simulink model "Demo"  (R2021a)
settings: Solver=FixedStepDiscrete  StartTime=0.0  StopTime=10  FixedStep=0.005  RelTol=1e-3  EnableMultiTasking=on
PreLoadFcn:
  | disp(pwd)
PostLoadFcn:
  | c2000demoscallback(1)
undefined symbols (not defined in the file or in its folder): CommandConstEnable, CommandData, FrameData, MailBoxRx, MailBoxTx, SCIAReceivedComplete, StatusConstClose, StatusConstClosed, StatusConstError, StatusConstHoming, StatusConstIdle, StatusConstPaused, StatusConstReady, StatusConstReset, StatusConstRunning, StatusConstStart, StatusConstStopped, StatusData
libraries: simulink x28, c280xlib x19, idelinklib_common x16, c2000lib x1, pid_lib x1, c2833xlib x1
(part 2 of 3)

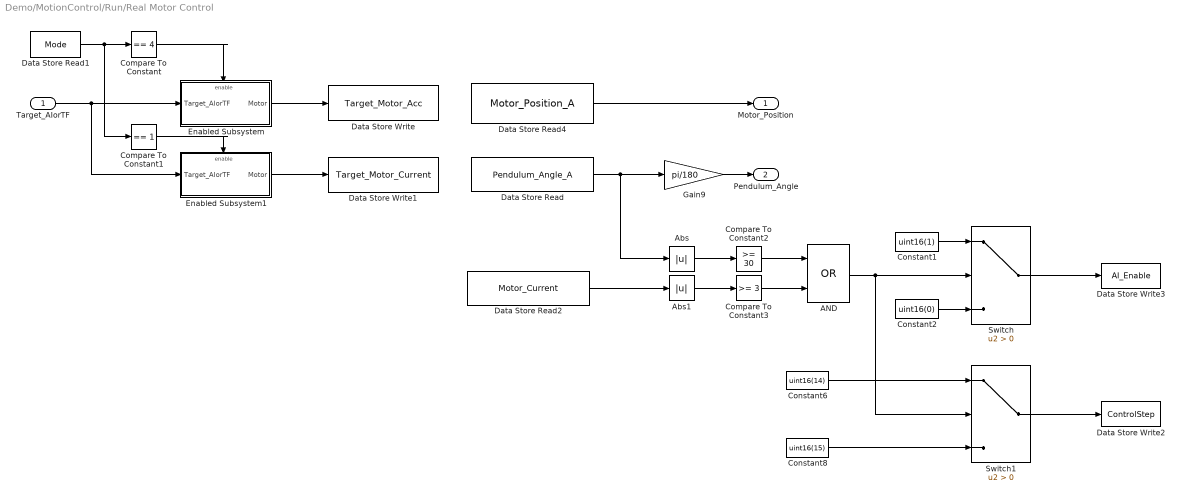
== system Demo/MotionControl/Run/Real Motor Control ==
  Target_AIorTF : Inport
  AND : Logic  Operator=OR  AllPortsSameDT=off  OutDataTypeStr=boolean
  Abs : Abs
  Abs1 : Abs
  Compare To Constant : simulink/Logic and Bit Operations/Compare To Constant  relop===  const=4  OutDataTypeStr=boolean
  Compare To Constant1 : simulink/Logic and Bit Operations/Compare To Constant  relop===  const=1  OutDataTypeStr=boolean
  Compare To Constant2 : simulink/Logic and Bit Operations/Compare To Constant  relop=>=  const=30  OutDataTypeStr=boolean
  Compare To Constant3 : simulink/Logic and Bit Operations/Compare To Constant  relop=>=  const=3  OutDataTypeStr=boolean
  Constant1 : Constant  Value=uint16(1)
  Constant2 : Constant  Value=uint16(0)
  Constant6 : Constant  Value=uint16(14)
  Constant8 : Constant  Value=uint16(15)
  Data Store Read : DataStoreRead  DataStoreName=Pendulum_Angle_A  IndexOptions=Index vector (dialog)  Indices=1  OutputSizes=1
  Data Store Read1 : DataStoreRead  DataStoreName=Mode  IndexOptions=Index vector (dialog)  Indices=1  OutputSizes=1
  Data Store Read2 : DataStoreRead  DataStoreName=Motor_Current  IndexOptions=Index vector (dialog)  Indices=1  OutputSizes=1
  Data Store Read4 : DataStoreRead  DataStoreName=Motor_Position_A  IndexOptions=Index vector (dialog)  Indices=1  OutputSizes=1
  Data Store Write : DataStoreWrite  DataStoreName=Target_Motor_Acc  IndexOptions=Index vector (dialog)  Indices=1  OutputSizes=1
  Data Store Write1 : DataStoreWrite  DataStoreName=Target_Motor_Current  IndexOptions=Index vector (dialog)  Indices=1  OutputSizes=1
  Data Store Write2 : DataStoreWrite  DataStoreName=ControlStep  IndexOptions=Index vector (dialog)  Indices=1  OutputSizes=1
  Data Store Write3 : DataStoreWrite  DataStoreName=AI_Enable  IndexOptions=Index vector (dialog)  Indices=1  OutputSizes=1
  Enabled Subsystem : Subsystem  TreatAsAtomicUnit=on
  Enabled Subsystem1 : Subsystem  TreatAsAtomicUnit=on
  Gain9 : Gain  Gain=pi/180  OutDataTypeStr=double
  Switch : Switch  Criteria=u2 > Threshold
  Switch1 : Switch  Criteria=u2 > Threshold
  Motor_Position : Outport  VectorParamsAs1DForOutWhenUnconnected=off
  Pendulum_Angle : Outport  Port=2  VectorParamsAs1DForOutWhenUnconnected=off
  wires:
  Compare To Constant1/1 -> Enabled Subsystem1/Enable
  Enabled Subsystem1/1(Motor) -> Data Store Write1/1
  Enabled Subsystem/1(Motor) -> Data Store Write/1
  Compare To Constant/1 -> Enabled Subsystem/Enable
  Data Store Read1/1 -> Compare To Constant/1, Compare To Constant1/1
  Target_AIorTF/1 -> Enabled Subsystem/1(Target_AIorTF), Enabled Subsystem1/1(Target_AIorTF)
  Gain9/1 -> Pendulum_Angle/1
  Data Store Read4/1 -> Motor_Position/1
  Compare To Constant2/1 -> AND/1
  Compare To Constant3/1 -> AND/2
  AND/1 -> Switch1/2, Switch/2
  Constant8/1 -> Switch1/3
  Data Store Read2/1 -> Abs1/1
  Abs1/1 -> Compare To Constant3/1
  Constant2/1 -> Switch/3
  Constant6/1 -> Switch1/1
  Abs/1 -> Compare To Constant2/1
  Data Store Read/1 -> Abs/1, Gain9/1
  Switch/1 -> Data Store Write3/1
  Switch1/1 -> Data Store Write2/1
  Constant1/1 -> Switch/1

== system Demo/MotionControl/Start/BG ==
  Action Port : ActionPort  ActionPortLabel=case [ 3 ]:
  BG : Constant  Value=[hex2dec('4742') 0 0 0]  OutDataTypeStr=uint16
  Constant : Constant  Value=uint16(15)  SampleTime=-1
  Data Store Write2 : DataStoreWrite  DataStoreName=ControlStep  IndexOptions=Index vector (dialog)  Indices=1  OutputSizes=1
  eCANA Transmit : Subsystem  TreatAsAtomicUnit=on  mask(eCANA Transimit Blocks){MailBoxTx=1, MailBoxRx=4}
      mask help: eCANA MailBox Transimit
      mask DialogControl ParameterGroup Prompt: Parameter Setting
  wires:
  BG/1 -> eCANA Transmit/1(DataTx)
  Constant/1 -> Data Store Write2/1

== system Demo/MotionControl/Start/MO=1 ==
  Action Port : ActionPort  ActionPortLabel=case [ 1 ]:
  Add Constant : Bias  Bias=uint16(1)
  Data Store Read : DataStoreRead  DataStoreName=ControlStep  IndexOptions=Index vector (dialog)  Indices=1  OutputSizes=1
  Data Store Write1 : DataStoreWrite  DataStoreName=ControlStep  IndexOptions=Index vector (dialog)  Indices=1  OutputSizes=1
  Delay500ms : Subsystem  mask(System Outputs){ShowInLibBrowser=0}
      mask prompts: ShowInLibBrowser "Simulink:masks:CustCodeMaskParam1_MP"
      settings: CopyFcn=cccopyfcn(gcb)  OpenFcn=ccopenfcn('System Outputs Function')
      mask Help: eval('feval(''rtwprivate'',''rtwhelpview'',''rtw_sys_outputs_block'')');
      mask Display: disp('System\nOutputs');
  MO : Constant  Value=[hex2dec('4F4D') 0 1 0]  OutDataTypeStr=uint16
  eCANA Transmit : Subsystem  TreatAsAtomicUnit=on  mask(eCANA Transimit Blocks){MailBoxTx=1, MailBoxRx=4}
      mask help: eCANA MailBox Transimit
      mask DialogControl ParameterGroup Prompt: Parameter Setting
  wires:
  Add Constant/1 -> Data Store Write1/1
  MO/1 -> eCANA Transmit/1(DataTx)
  Data Store Read/1 -> Add Constant/1

== system Demo/MotionControl/Start/UM=1or4 ==
  Action Port : ActionPort  ActionPortLabel=case [ 2 ]:
  Add Constant : Bias  Bias=uint16(1)
  Constant : Constant  Value=hex2dec('4D55')  OutDataTypeStr=uint16
  Constant1 : Constant  Value=uint16(0)
  Constant2 : Constant  Value=uint16(0)
  Constant3 : Constant  Value=uint16(1)
  Constant4 : Constant  Value=uint16(4)
  Data Store Read : DataStoreRead  DataStoreName=ControlStep  IndexOptions=Index vector (dialog)  Indices=1  OutputSizes=1
  Data Store Read1 : DataStoreRead  DataStoreName=CommandData  IndexOptions=Index vector (dialog)  Indices=1  OutputSizes=1
  Data Store Write1 : DataStoreWrite  DataStoreName=ControlStep  IndexOptions=Index vector (dialog)  Indices=1  OutputSizes=1
  Data Store Write2 : DataStoreWrite  DataStoreName=Mode  IndexOptions=Index vector (dialog)  Indices=1  OutputSizes=1
  Mux : Mux
  Selector : Selector  InputPortWidth=8  IndexOptions=Index vector (dialog)  Indices=1  OutputSizes=1
  Switch : Switch  Criteria=u2 > Threshold
  eCANA Transmit : Subsystem  TreatAsAtomicUnit=on  mask(eCANA Transimit Blocks){MailBoxTx=1, MailBoxRx=4}
      mask help: eCANA MailBox Transimit
      mask DialogControl ParameterGroup Prompt: Parameter Setting
  wires:
  Add Constant/1 -> Data Store Write1/1
  Data Store Read/1 -> Add Constant/1
  Constant2/1 -> Mux/4
  Data Store Read1/1 -> Selector/1
  Constant3/1 -> Switch/1
  Constant4/1 -> Switch/3
  Constant/1 -> Mux/1
  Constant1/1 -> Mux/2
  Mux/1 -> eCANA Transmit/1(DataTx)
  Selector/1 -> Switch/2
  Switch/1 -> Data Store Write2/1, Mux/3

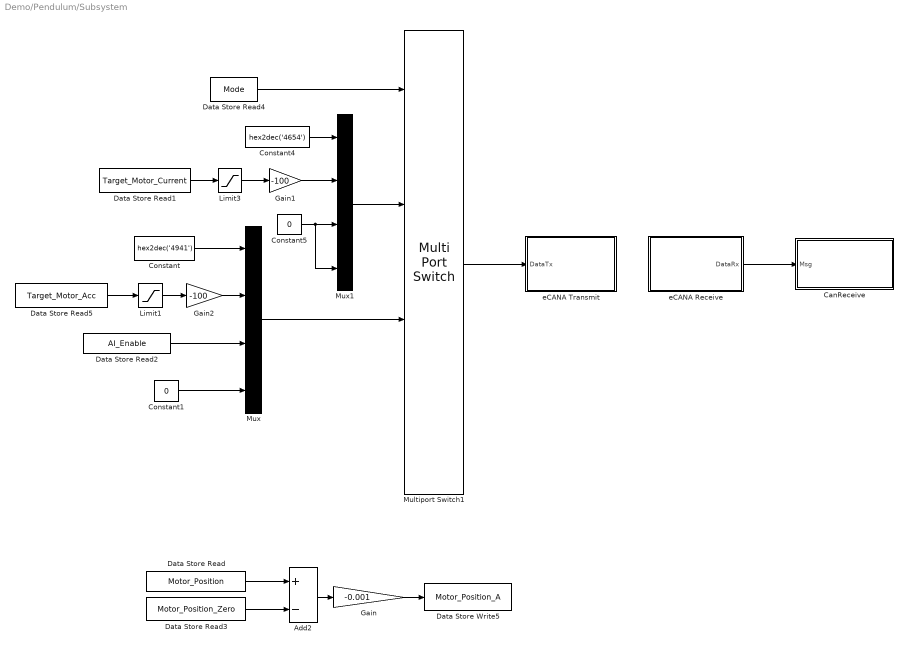
== system Demo/Pendulum/Subsystem ==
  Add2 : Sum  Inputs=+-
  CanReceive : Subsystem  TreatAsAtomicUnit=on
  Constant : Constant  Value=hex2dec('4941')  OutDataTypeStr=uint16
  Constant1 : Constant  Value=0  OutDataTypeStr=uint16
  Constant4 : Constant  Value=hex2dec('4654')  OutDataTypeStr=uint16
  Constant5 : Constant  Value=0  OutDataTypeStr=uint16
  Data Store Read : DataStoreRead  DataStoreName=Motor_Position  IndexOptions=Index vector (dialog)  Indices=1  OutputSizes=1
  Data Store Read1 : DataStoreRead  DataStoreName=Target_Motor_Current  IndexOptions=Index vector (dialog)  Indices=1  OutputSizes=1
  Data Store Read2 : DataStoreRead  DataStoreName=AI_Enable  IndexOptions=Index vector (dialog)  Indices=1  OutputSizes=1
  Data Store Read3 : DataStoreRead  DataStoreName=Motor_Position_Zero  IndexOptions=Index vector (dialog)  Indices=1  OutputSizes=1
  Data Store Read4 : DataStoreRead  DataStoreName=Mode  IndexOptions=Index vector (dialog)  Indices=1  OutputSizes=1
  Data Store Read5 : DataStoreRead  DataStoreName=Target_Motor_Acc  IndexOptions=Index vector (dialog)  Indices=1  OutputSizes=1
  Data Store Write5 : DataStoreWrite  DataStoreName=Motor_Position_A  IndexOptions=Index vector (dialog)  Indices=1  OutputSizes=1
  Gain : Gain  Gain=-0.001
  Gain1 : Gain  Gain=-100  OutDataTypeStr=uint16
  Gain2 : Gain  Gain=-100  OutDataTypeStr=uint16
  Limit1 : Saturate  UpperLimit=300  LowerLimit=-300
  Limit3 : Saturate  UpperLimit=3  LowerLimit=-3
  Multiport Switch1 : MultiPortSwitch  DataPortOrder=Specify indices  DataPortIndices={1,4}  DataPortForDefault=Additional data port  DiagnosticForDefault=None
  Mux : Mux
  Mux1 : Mux
  eCANA Receive : Subsystem  TreatAsAtomicUnit=on  mask(eCANA Transimit Blocks){MailBoxTx=1, MailBoxRx=4}
      mask help: eCANA MailBox Transimit
      mask DialogControl ParameterGroup Prompt: Parameter Setting
  eCANA Transmit : Subsystem  TreatAsAtomicUnit=on  mask(eCANA Transimit Blocks){MailBoxTx=1, MailBoxRx=4}
      mask help: eCANA MailBox Transimit
      mask DialogControl ParameterGroup Prompt: Parameter Setting
  wires:
  Data Store Read1/1 -> Limit3/1
  Data Store Read4/1 -> Multiport Switch1/1
  Constant4/1 -> Mux1/1
  Constant5/1 -> Mux1/4, Mux1/3
  Constant1/1 -> Mux/4
  Constant/1 -> Mux/1
  Data Store Read5/1 -> Limit1/1
  Gain/1 -> Data Store Write5/1
  Data Store Read3/1 -> Add2/2
  Add2/1 -> Gain/1
  Data Store Read/1 -> Add2/1
  Gain2/1 -> Mux/2
  Gain1/1 -> Mux1/2
  Mux/1 -> Multiport Switch1/3
  Mux1/1 -> Multiport Switch1/2
  Multiport Switch1/1 -> eCANA Transmit/1(DataTx)
  eCANA Receive/1(DataRx) -> CanReceive/1(Msg)
  Data Store Read2/1 -> Mux/3
  Limit1/1 -> Gain2/1
  Limit3/1 -> Gain1/1

== system Demo/Pendulum/Subsystem1 ==
  Add : Sum  Inputs=+-
  Data Store Read1 : DataStoreRead  DataStoreName=Pendulum_Angle_Zero  IndexOptions=Index vector (dialog)  Indices=1  OutputSizes=1
  Data Store Write1 : DataStoreWrite  DataStoreName=Pendulum_Angle_A  IndexOptions=Index vector (dialog)  Indices=1  OutputSizes=1
  Data Store Write2 : DataStoreWrite  DataStoreName=Pendulum_Angle  IndexOptions=Index vector (dialog)  Indices=1  OutputSizes=1
  Gain1 : Gain  Gain=360/10000  OutDataTypeStr=double
  eQEP : c280xlib/eQEP  useModule=eQEP1  pcInputmode=Quadrature-count  externalClockrate=2x resolution: Count the rising/falling edge  swapPolarityselection=Counterclockwise  qdfOutputport=off  qapPolarityselection=off  qbpPolarityselection=off  qipPolarityselection=off  qspPolarityselection=off  igatePolarityselection=off  sampleTime=-1  pcOutputport=on  pcMaximumvalue=4294967295  indexInitializationcheck=off  indexInitializationevent=Rising edge  strobeInitializationcheck=off  strobeInitializationevent=Rising edge  softwareInitializationcheck=on  softwareInitializationsource=Set to init value at start up  softwareInitializationmode=on  pcInitialvalue=4294962296  pcResetmode=Reset on the maximum position  ieloutputport=off  indexEventlatch=Rising edge  seloutputport=off  strobeEventlatch=Rising edge  pcefOutputport=off  enableEqepcapture=off  qctmrOutputport=off  qcprdOutputport=off  captureTimerprescaler=128  upEventprescaler=128  overflowErrorflag=off  directionErrorflag=off  captureTimerposition=On position counter read  unitTimerperiod=100000000  captureTimerlatch=off  capturePeriodlatch=off  positionCounterlatch=off  soenPolarityselection=off  spselPolarityselection=Index pin is used for sync output  compareValuesource=Specify via dialog  shadowMode=Load on QPOSCNT=0  compareValue=4294967295  syncOutputwidth=1  polaritySyncoutput=Active high  watchdogEnable=off  watchdogTimer=65535  outport1Datatype=auto  outport2Datatype=int32  outport3Datatype=auto  outport4Datatype=auto  outport5Datatype=auto  outport6Datatype=auto  outport7Datatype=auto  outport8Datatype=auto  outport9Datatype=auto  outport10Datatype=auto  outport11Datatype=auto  outport12Datatype=auto  eqepinterrupt_pce=off  eqepinterrupt_qpe=off  eqepinterrupt_qdc=off  eqepinterrupt_wto=off  eqepinterrupt_pcu=off  eqepinterrupt_pco=off  eqepinterrupt_pcr=off  eqepinterrupt_pcm=off  eqepinterrupt_sel=off  eqepinterrupt_iel=off  eqepinterrupt_uto=off  pheOutputport=off  watchdogOutputport=off  outport13Datatype=auto  outport14Datatype=auto
      settings: SourceProductName=Embedded Coder Support Package for Texas Instruments C2000 Processors
  wires:
  Data Store Read1/1 -> Add/2
  Gain1/1 -> Add/1, Data Store Write2/1
  eQEP/1 -> Gain1/1
  Add/1 -> Data Store Write1/1

== system Demo/Status Display/Enabled Subsystem ==
  Status1 : Inport
  Status2 : Inport  Port=2
  Enable : EnablePort
  Status Display : Subsystem  Commented=on  TreatAsAtomicUnit=on
  Status Display1 : Subsystem  TreatAsAtomicUnit=on
  Status Display2 : Subsystem  TreatAsAtomicUnit=on
  System Outputs1 : Subsystem  mask(System Outputs){ShowInLibBrowser=0}
      mask prompts: ShowInLibBrowser "Simulink:masks:CustCodeMaskParam1_MP"
      settings: CopyFcn=cccopyfcn(gcb)  OpenFcn=ccopenfcn('System Outputs Function')
      mask Help: eval('feval(''rtwprivate'',''rtwhelpview'',''rtw_sys_outputs_block'')');
      mask Display: disp('System\nOutputs');
  wires:
  Status1/1 -> Status Display/1(SEG), Status Display1/1(String)
  Status2/1 -> Status Display2/1(String)

== system Demo/Status Upload/PositionFloatToInt ==
  In1 : Inport
  Demux : Demux  Outputs=8
  MATLAB Function1 : MATLAB Function  TreatAsAtomicUnit=on
  MATLAB Function2 : MATLAB Function  TreatAsAtomicUnit=on
  MATLAB Function3 : MATLAB Function  TreatAsAtomicUnit=on
  MATLAB Function4 : MATLAB Function  TreatAsAtomicUnit=on
  MATLAB Function5 : MATLAB Function  TreatAsAtomicUnit=on
  MATLAB Function6 : MATLAB Function  TreatAsAtomicUnit=on
  MATLAB Function7 : MATLAB Function  TreatAsAtomicUnit=on
  MATLAB Function8 : MATLAB Function  TreatAsAtomicUnit=on
  Mux : Mux  Inputs=8
  Subsystem : Subsystem  Commented=on
  Out1 : Outport
  wires:
  Demux/5 -> MATLAB Function5/1(u)
  Demux/2 -> MATLAB Function2/1(u)
  Demux/1 -> MATLAB Function1/1(u)
  Demux/6 -> MATLAB Function6/1(u)
  MATLAB Function4/1(y) -> Mux/4
  Demux/4 -> MATLAB Function4/1(u)
  MATLAB Function3/1(y) -> Mux/3
  Demux/3 -> MATLAB Function3/1(u)
  MATLAB Function6/1(y) -> Mux/6
  MATLAB Function1/1(y) -> Mux/1
  MATLAB Function5/1(y) -> Mux/5
  MATLAB Function2/1(y) -> Mux/2
  Mux/1 -> Out1/1
  Demux/7 -> MATLAB Function7/1(u)
  Demux/8 -> MATLAB Function8/1(u)
  MATLAB Function7/1(y) -> Mux/7
  MATLAB Function8/1(y) -> Mux/8
  In1/1 -> Demux/1

== system Demo/Status Upload/Subsystem3 ==
  In1 : Inport
  Add : Sum  Inputs=++++++++++++++++
  Demux : Demux  Outputs=8
  Demux{1..8} (8 alike) : Demux  Outputs=2
  Out1 : Outport
  wires:
  In1/1 -> Demux/1
  Demux/1 -> Demux1/1
  Demux/2 -> Demux2/1
  Demux/6 -> Demux6/1
  Demux/5 -> Demux5/1
  Demux/4 -> Demux4/1
  Demux/3 -> Demux3/1
  Demux1/1 -> Add/1
  Demux1/2 -> Add/2
  Demux2/1 -> Add/3
  Demux2/2 -> Add/4
  Demux6/2 -> Add/12
  Demux3/1 -> Add/5
  Demux3/2 -> Add/6
  Demux4/1 -> Add/7
  Demux4/2 -> Add/8
  Demux5/1 -> Add/9
  Demux5/2 -> Add/10
  Demux6/1 -> Add/11
  Add/1 -> Out1/1
  Demux/7 -> Demux7/1
  Demux/8 -> Demux8/1
  Demux7/1 -> Add/13
  Demux7/2 -> Add/14
  Demux8/1 -> Add/15
  Demux8/2 -> Add/16

== system Demo/Status Upload/VariantSubsystem ==
  note: 1) Add Subsystem or Model blocks as valid variant choices.
      | 2) You cannot connect blocks at this level. At simulation, connectivity is automatically
      | determined, based on the active variant and port name matching.
  In1 : Inport
  Send10 : Subsystem  TreatAsAtomicUnit=on  VariantControl=Variant2
      settings: RTWSystemCode=Nonreusable function
  Srnd4 : Subsystem  TreatAsAtomicUnit=on  VariantControl=Variant1
      settings: RTWSystemCode=Nonreusable function

== system Demo/System Config/CAN_Config_C ==
  Model Header : Subsystem  mask(Model Header){ShowInLibBrowser=0}
      mask prompts: ShowInLibBrowser "Simulink:masks:CustCodeMaskParam1_MP"
      settings: CopyFcn=cccopyfcn(gcb)  OpenFcn=ccopenfcn('Model Header')
      mask Help: eval('feval(''rtwprivate'',''rtwhelpview'',''rtw_model_header_block'')');
      mask Display: disp('Model\nHeader');
  Model Source1 : Subsystem  mask(Model Source){ShowInLibBrowser=0}
      mask prompts: ShowInLibBrowser "Simulink:masks:CustCodeMaskParam1_MP"
      settings: CopyFcn=cccopyfcn(gcb)  OpenFcn=ccopenfcn('Model Source')
      mask Help: eval('feval(''rtwprivate'',''rtwhelpview'',''rtw_model_source_block'')');
      mask Display: disp('Model\nSource');
  System Initialize1 : Subsystem  mask(System Initialize){ShowInLibBrowser=0}
      mask prompts: ShowInLibBrowser "Simulink:masks:CustCodeMaskParam1_MP"
      settings: CopyFcn=cccopyfcn(gcb)  OpenFcn=ccopenfcn('System Initialize Function')
      mask Help: eval('feval(''rtwprivate'',''rtwhelpview'',''rtw_sys_initialize_block'')');
      mask Display: disp('System\nInitialize');

== system Demo/System Config/CAN_Config_S ==
  note: CAN 邮箱号说明
      | A B
      | 0：广播命令 0：广播命令1：ID1发送 1：ID4发送
      | 2：ID2发送 2：ID5发送
      | 3：ID3发送 3：ID6发送
      | 4：ID1接收 4：ID4接收
      | 5：ID2接收 5：ID5接收
      | 6：ID3接收 6：ID6接收
  Constant : Constant  Value=false
  Model Header : Subsystem  Commented=on  mask(Model Header){ShowInLibBrowser=0}
      mask prompts: ShowInLibBrowser "Simulink:masks:CustCodeMaskParam1_MP"
      settings: CopyFcn=cccopyfcn(gcb)  OpenFcn=ccopenfcn('Model Header')
      mask Help: eval('feval(''rtwprivate'',''rtwhelpview'',''rtw_model_header_block'')');
      mask DialogControl ShowInLibBrowser Prompt: Mask Parameter 1:
      mask Display: disp('Model\nHeader');
  Model Source1 : Subsystem  mask(Model Source){ShowInLibBrowser=0}
      mask prompts: ShowInLibBrowser "Simulink:masks:CustCodeMaskParam1_MP"
      settings: CopyFcn=cccopyfcn(gcb)  OpenFcn=ccopenfcn('Model Source')
      mask Help: eval('feval(''rtwprivate'',''rtwhelpview'',''rtw_model_source_block'')');
      mask DialogControl ShowInLibBrowser Prompt: Mask Parameter 1:
      mask Display: disp('Model\nSource');
  Subsystem : Subsystem
  System Initialize1 : Subsystem  Commented=on  mask(System Initialize){ShowInLibBrowser=0}
      mask prompts: ShowInLibBrowser "Simulink:masks:CustCodeMaskParam1_MP"
      settings: CopyFcn=cccopyfcn(gcb)  OpenFcn=ccopenfcn('System Initialize Function')
      mask Help: eval('feval(''rtwprivate'',''rtwhelpview'',''rtw_sys_initialize_block'')');
      mask DialogControl ShowInLibBrowser Prompt: Mask Parameter 1:
      mask Display: disp('System\nInitialize');
  eCANA Transmit1 : Subsystem  Commented=on  TreatAsAtomicUnit=on  mask(eCANA Transimit Blocks){MailBox=1}
      mask help: eCANA MailBox Transimit
      mask DialogControl ParameterGroup Prompt: Parameter Setting
  eCANA Transmit2 : Subsystem  Commented=on  TreatAsAtomicUnit=on  mask(eCANA Transimit Blocks){MailBox=2}
      mask help: eCANA MailBox Transimit
      mask DialogControl ParameterGroup Prompt: Parameter Setting
  eCANA Transmit3 : Subsystem  Commented=on  TreatAsAtomicUnit=on  mask(eCANA Transimit Blocks){MailBox=3}
      mask help: eCANA MailBox Transimit
      mask DialogControl ParameterGroup Prompt: Parameter Setting
  eCANB Transmit1 : Subsystem  Commented=on  TreatAsAtomicUnit=on  mask(eCANB Transimit Blocks){MailBox=1}
      mask help: eCANB MailBox Transimit
      mask DialogControl ParameterGroup Prompt: Parameter Setting
  eCANB Transmit2 : Subsystem  Commented=on  TreatAsAtomicUnit=on  mask(eCANB Transimit Blocks){MailBox=2}
      mask help: eCANB MailBox Transimit
      mask DialogControl ParameterGroup Prompt: Parameter Setting
  eCANB Transmit3 : Subsystem  Commented=on  TreatAsAtomicUnit=on  mask(eCANB Transimit Blocks){MailBox=3}
      mask help: eCANB MailBox Transimit
      mask DialogControl ParameterGroup Prompt: Parameter Setting
  wires:
  Constant/1 -> Subsystem/Enable

== system Demo/System Config/HC595_Config ==
  Model Header : Subsystem  mask(Model Header){ShowInLibBrowser=0}
      mask prompts: ShowInLibBrowser "Simulink:masks:CustCodeMaskParam1_MP"
      settings: CopyFcn=cccopyfcn(gcb)  OpenFcn=ccopenfcn('Model Header')
      mask Help: eval('feval(''rtwprivate'',''rtwhelpview'',''rtw_model_header_block'')');
      mask Display: disp('Model\nHeader');
  Model Source : Subsystem  mask(Model Source){ShowInLibBrowser=0}
      mask prompts: ShowInLibBrowser "Simulink:masks:CustCodeMaskParam1_MP"
      settings: CopyFcn=cccopyfcn(gcb)  OpenFcn=ccopenfcn('Model Source')
      mask Help: eval('feval(''rtwprivate'',''rtwhelpview'',''rtw_model_source_block'')');
      mask Display: disp('Model\nSource');
  System Initialize1 : Subsystem  mask(System Initialize){ShowInLibBrowser=0}
      mask prompts: ShowInLibBrowser "Simulink:masks:CustCodeMaskParam1_MP"
      settings: CopyFcn=cccopyfcn(gcb)  OpenFcn=ccopenfcn('System Initialize Function')
      mask Help: eval('feval(''rtwprivate'',''rtwhelpview'',''rtw_sys_initialize_block'')');
      mask Display: disp('System\nInitialize');

== system Demo/System Config/LCD_Config ==
  Model Header : Subsystem  Commented=on  mask(Model Header){ShowInLibBrowser=0}
      mask prompts: ShowInLibBrowser "Simulink:masks:CustCodeMaskParam1_MP"
      settings: CopyFcn=cccopyfcn(gcb)  OpenFcn=ccopenfcn('Model Header')
      mask Help: eval('feval(''rtwprivate'',''rtwhelpview'',''rtw_model_header_block'')');
      mask Display: disp('Model\nHeader');
  Model Source : Subsystem  mask(Model Source){ShowInLibBrowser=0}
      mask prompts: ShowInLibBrowser "Simulink:masks:CustCodeMaskParam1_MP"
      settings: CopyFcn=cccopyfcn(gcb)  OpenFcn=ccopenfcn('Model Source')
      mask Help: eval('feval(''rtwprivate'',''rtwhelpview'',''rtw_model_source_block'')');
      mask Display: disp('Model\nSource');
  System Initialize : Subsystem  mask(System Initialize){ShowInLibBrowser=0}
      mask prompts: ShowInLibBrowser "Simulink:masks:CustCodeMaskParam1_MP"
      settings: CopyFcn=cccopyfcn(gcb)  OpenFcn=ccopenfcn('System Initialize Function')
      mask Help: eval('feval(''rtwprivate'',''rtwhelpview'',''rtw_sys_initialize_block'')');
      mask Display: disp('System\nInitialize');

== system Demo/System Config/SCI_Config ==
  Model Header : Subsystem  mask(Model Header){ShowInLibBrowser=0}
      mask prompts: ShowInLibBrowser "Simulink:masks:CustCodeMaskParam1_MP"
      settings: CopyFcn=cccopyfcn(gcb)  OpenFcn=ccopenfcn('Model Header')
      mask Help: eval('feval(''rtwprivate'',''rtwhelpview'',''rtw_model_header_block'')');
      mask Display: disp('Model\nHeader');
  Model Source : Subsystem  mask(Model Source){ShowInLibBrowser=0}
      mask prompts: ShowInLibBrowser "Simulink:masks:CustCodeMaskParam1_MP"
      settings: CopyFcn=cccopyfcn(gcb)  OpenFcn=ccopenfcn('Model Source')
      mask Help: eval('feval(''rtwprivate'',''rtwhelpview'',''rtw_model_source_block'')');
      mask Display: disp('Model\nSource');

== system Demo/Command Download/SCIA_RX_Process/Process ==
  Compare To Constant : simulink/Logic and Bit Operations/Compare To Constant  relop===  const=uint8(1)  OutDataTypeStr=boolean
  Constant : Constant  Value=SCIAReceivedComplete  OutDataTypeStr=uint16  SampleTime=-1
  Enabled Subsystem : Subsystem  TreatAsAtomicUnit=on
  System Outputs : Subsystem  mask(System Outputs){ShowInLibBrowser=0}
      mask prompts: ShowInLibBrowser "Simulink:masks:CustCodeMaskParam1_MP"
      settings: CopyFcn=cccopyfcn(gcb)  OpenFcn=ccopenfcn('System Outputs Function')
      mask Help: eval('feval(''rtwprivate'',''rtwhelpview'',''rtw_sys_outputs_block'')');
      mask Display: disp('System\nOutputs');
  wires:
  Constant/1 -> Compare To Constant/1
  Compare To Constant/1 -> Enabled Subsystem/Enable

== system Demo/Command Download/SCIA_RX_Process/Receive ==
  SCIAReceive : c280xlib/SCI Receive  sciModule=A  dataHead=''  dataTail=''  dataType=uint16  dataDim=1  initValue=0  errOption=Output the last received value  errValue=0  sampleTime=-1  outputStatus=off  postInterrupt=on  numFifo=1
      settings: SourceProductBaseCode=TIC2000
  wires:
  SCIAReceive/1 -> ?  "SCIAReceivedByte"

== system Demo/MotionControl/Close/eCANA Transmit/System Outputs ==

== system Demo/MotionControl/Home/TForAI1/Enabled Subsystem ==
  Target_AIorTF : Inport
  Enable : EnablePort
  Motor : Outport
  wires:
  Target_AIorTF/1 -> Motor/1

== system Demo/MotionControl/Home/TForAI1/Enabled Subsystem1 ==
  Target_AIorTF : Inport
  Enable : EnablePort
  Motor : Outport
  wires:
  Target_AIorTF/1 -> Motor/1

== system Demo/MotionControl/Reset/AI=0/eCANA Transmit ==
  DataTx : Inport
  Bus Assignment : BusAssignment  Priority=1  AssignedSignals=TxWord
  Data Store Read : DataStoreRead  DataStoreName=CanMsgA  IndexOptions=Index vector (dialog)  Indices=1  OutputSizes=1
  Data Store Write : DataStoreWrite  DataStoreName=CanMsgA  IndexOptions=Index vector (dialog)  Indices=1  OutputSizes=1
  System Outputs : Subsystem  Priority=2  mask(System Outputs){MailBox=0}
      settings: CopyFcn=cccopyfcn(gcb)  OpenFcn=ccopenfcn('System Outputs Function')
      mask Help: eval('feval(''rtwprivate'',''rtwhelpview'',''rtw_sys_outputs_block'')');
      mask TypeOptions MailBox: 0 | 1 | 2 | 3 | 4 | 5
  wires:
  Bus Assignment/1 -> Data Store Write/1
  Data Store Read/1 -> Bus Assignment/1
  DataTx/1 -> Bus Assignment/2

== system Demo/MotionControl/Reset/AI=1/Subsystem1 ==
  In1 : Inport
  In2 : Inport  Port=2
  In3 : Inport  Port=3
  Enable : EnablePort
  Add : Sum
  Add Constant : Bias  Bias=uint16(1)
  Data Store Read : DataStoreRead  DataStoreName=ControlStep  IndexOptions=Index vector (dialog)  Indices=1  OutputSizes=1
  Data Store Write : DataStoreWrite  DataStoreName=Motor_Current  IndexOptions=Index vector (dialog)  Indices=1  OutputSizes=1
  Data Store Write1 : DataStoreWrite  DataStoreName=Motor_Position  IndexOptions=Index vector (dialog)  Indices=1  OutputSizes=1
  Data Store Write2 : DataStoreWrite  DataStoreName=ControlStep  IndexOptions=Index vector (dialog)  Indices=1  OutputSizes=1
  Data Type Conversion : DataTypeConversion  OutDataTypeStr=int32
  Data Type Conversion2 : DataTypeConversion  OutDataTypeStr=int32
  Gain2 : Gain  Gain=0.001  OutDataTypeStr=double
  Shift Arithmetic1 : ArithShift  BitShiftNumber=16  BitShiftDirection=Left
  Switch : Switch  Criteria=u2 > Threshold  Threshold=2
  wires:
  Data Type Conversion/1 -> Add/1
  Data Type Conversion2/1 -> Shift Arithmetic1/1
  Add/1 -> Gain2/1
  Gain2/1 -> Data Store Write1/1
  Shift Arithmetic1/1 -> Add/2
  In1/1 -> Switch/2, Data Store Write/1
  In2/1 -> Data Type Conversion/1
  In3/1 -> Data Type Conversion2/1
  Data Store Read/1 -> Switch/3, Add Constant/1
  Add Constant/1 -> Switch/1
  Switch/1 -> Data Store Write2/1

== system Demo/MotionControl/Reset/AI=1/eCANA Receive ==
  Bus Selector : BusSelector  Priority=3  OutputSignals=RxWord
  Data Store Read1 : DataStoreRead  DataStoreName=CanMsgA  IndexOptions=Index vector (dialog)  Indices=1  OutputSizes=1
  System Outputs : Subsystem  Priority=2  mask(System Outputs){MailBox=0}
      settings: CopyFcn=cccopyfcn(gcb)  OpenFcn=ccopenfcn('System Outputs Function')
      mask Help: eval('feval(''rtwprivate'',''rtwhelpview'',''rtw_sys_outputs_block'')');
      mask TypeOptions MailBox: 0 | 1 | 2 | 3 | 4 | 5
  DataRx : Outport
  wires:
  Bus Selector/1 -> DataRx/1  "<RxWord>"
  Data Store Read1/1 -> Bus Selector/1

== system Demo/MotionControl/Reset/AI=1/eCANA Transmit ==
  DataTx : Inport
  Bus Assignment : BusAssignment  Priority=1  AssignedSignals=TxWord
  Data Store Read : DataStoreRead  DataStoreName=CanMsgA  IndexOptions=Index vector (dialog)  Indices=1  OutputSizes=1
  Data Store Write : DataStoreWrite  DataStoreName=CanMsgA  IndexOptions=Index vector (dialog)  Indices=1  OutputSizes=1
  System Outputs : Subsystem  Priority=2  mask(System Outputs){MailBox=0}
      settings: CopyFcn=cccopyfcn(gcb)  OpenFcn=ccopenfcn('System Outputs Function')
      mask Help: eval('feval(''rtwprivate'',''rtwhelpview'',''rtw_sys_outputs_block'')');
      mask TypeOptions MailBox: 0 | 1 | 2 | 3 | 4 | 5
  wires:
  DataTx/1 -> Bus Assignment/2
  Data Store Read/1 -> Bus Assignment/1
  Bus Assignment/1 -> Data Store Write/1

== system Demo/MotionControl/Reset/BG /eCANA Transmit ==
  DataTx : Inport
  Bus Assignment : BusAssignment  Priority=1  AssignedSignals=TxWord
  Data Store Read : DataStoreRead  DataStoreName=CanMsgA  IndexOptions=Index vector (dialog)  Indices=1  OutputSizes=1
  Data Store Write : DataStoreWrite  DataStoreName=CanMsgA  IndexOptions=Index vector (dialog)  Indices=1  OutputSizes=1
  System Outputs : Subsystem  Priority=2  mask(System Outputs){MailBox=0}
      settings: CopyFcn=cccopyfcn(gcb)  OpenFcn=ccopenfcn('System Outputs Function')
      mask Help: eval('feval(''rtwprivate'',''rtwhelpview'',''rtw_sys_outputs_block'')');
      mask TypeOptions MailBox: 0 | 1 | 2 | 3 | 4 | 5
  wires:
  DataTx/1 -> Bus Assignment/2
  Data Store Read/1 -> Bus Assignment/1
  Bus Assignment/1 -> Data Store Write/1

== system Demo/MotionControl/Reset/JV=0/eCANA Transmit ==
  DataTx : Inport
  Bus Assignment : BusAssignment  Priority=1  AssignedSignals=TxWord
  Data Store Read : DataStoreRead  DataStoreName=CanMsgA  IndexOptions=Index vector (dialog)  Indices=1  OutputSizes=1
  Data Store Write : DataStoreWrite  DataStoreName=CanMsgA  IndexOptions=Index vector (dialog)  Indices=1  OutputSizes=1
  System Outputs : Subsystem  Priority=2  mask(System Outputs){MailBox=0}
      settings: CopyFcn=cccopyfcn(gcb)  OpenFcn=ccopenfcn('System Outputs Function')
      mask Help: eval('feval(''rtwprivate'',''rtwhelpview'',''rtw_sys_outputs_block'')');
      mask TypeOptions MailBox: 0 | 1 | 2 | 3 | 4 | 5
  wires:
  Bus Assignment/1 -> Data Store Write/1
  Data Store Read/1 -> Bus Assignment/1
  DataTx/1 -> Bus Assignment/2

== system Demo/MotionControl/Reset/MO=0/Delay500ms ==

== system Demo/MotionControl/Reset/MO=0/eCANA Transmit ==
  DataTx : Inport
  Bus Assignment : BusAssignment  Priority=1  AssignedSignals=TxWord
  Data Store Read : DataStoreRead  DataStoreName=CanMsgA  IndexOptions=Index vector (dialog)  Indices=1  OutputSizes=1
  Data Store Write : DataStoreWrite  DataStoreName=CanMsgA  IndexOptions=Index vector (dialog)  Indices=1  OutputSizes=1
  System Outputs : Subsystem  Priority=2  mask(System Outputs){MailBox=0}
      settings: CopyFcn=cccopyfcn(gcb)  OpenFcn=ccopenfcn('System Outputs Function')
      mask Help: eval('feval(''rtwprivate'',''rtwhelpview'',''rtw_sys_outputs_block'')');
      mask TypeOptions MailBox: 0 | 1 | 2 | 3 | 4 | 5
  wires:
  Bus Assignment/1 -> Data Store Write/1
  Data Store Read/1 -> Bus Assignment/1
  DataTx/1 -> Bus Assignment/2

== system Demo/MotionControl/Reset/MO=1/Delay500ms ==

== system Demo/MotionControl/Reset/MO=1/eCANA Transmit ==
  DataTx : Inport
  Bus Assignment : BusAssignment  Priority=1  AssignedSignals=TxWord
  Data Store Read : DataStoreRead  DataStoreName=CanMsgA  IndexOptions=Index vector (dialog)  Indices=1  OutputSizes=1
  Data Store Write : DataStoreWrite  DataStoreName=CanMsgA  IndexOptions=Index vector (dialog)  Indices=1  OutputSizes=1
  System Outputs : Subsystem  Priority=2  mask(System Outputs){MailBox=0}
      settings: CopyFcn=cccopyfcn(gcb)  OpenFcn=ccopenfcn('System Outputs Function')
      mask Help: eval('feval(''rtwprivate'',''rtwhelpview'',''rtw_sys_outputs_block'')');
      mask TypeOptions MailBox: 0 | 1 | 2 | 3 | 4 | 5
  wires:
  DataTx/1 -> Bus Assignment/2
  Data Store Read/1 -> Bus Assignment/1
  Bus Assignment/1 -> Data Store Write/1

== system Demo/MotionControl/Reset/PX/eCANA Transmit ==
  DataTx : Inport
  Bus Assignment : BusAssignment  Priority=1  AssignedSignals=TxWord
  Data Store Read : DataStoreRead  DataStoreName=CanMsgA  IndexOptions=Index vector (dialog)  Indices=1  OutputSizes=1
  Data Store Write : DataStoreWrite  DataStoreName=CanMsgA  IndexOptions=Index vector (dialog)  Indices=1  OutputSizes=1
  System Outputs : Subsystem  Priority=2  mask(System Outputs){MailBox=0}
      settings: CopyFcn=cccopyfcn(gcb)  OpenFcn=ccopenfcn('System Outputs Function')
      mask Help: eval('feval(''rtwprivate'',''rtwhelpview'',''rtw_sys_outputs_block'')');
      mask TypeOptions MailBox: 0 | 1 | 2 | 3 | 4 | 5
  wires:
  DataTx/1 -> Bus Assignment/2
  Data Store Read/1 -> Bus Assignment/1
  Bus Assignment/1 -> Data Store Write/1

== system Demo/MotionControl/Reset/Set_P0/Enabled Subsystem ==
  int_L : Inport
  int_H : Inport  Port=2
  Enable : EnablePort
  Add : Sum  Commented=on
  Add1 : Sum  Inputs=+-
  Constant : Constant  Value=uint16(15)  SampleTime=-1
  Constant1 : Constant  Value=200
  Data Store Read : DataStoreRead  DataStoreName=Motor_Position  IndexOptions=Index vector (dialog)  Indices=1  OutputSizes=1
  Data Store Write : DataStoreWrite  DataStoreName=Motor_Position  IndexOptions=Index vector (dialog)  Indices=1  OutputSizes=1
  Data Store Write1 : DataStoreWrite  DataStoreName=Motor_Position_Zero  IndexOptions=Index vector (dialog)  Indices=1  OutputSizes=1
  Data Store Write2 : DataStoreWrite  DataStoreName=ControlStep  IndexOptions=Index vector (dialog)  Indices=1  OutputSizes=1
  Data Type Conversion : DataTypeConversion  Commented=on  OutDataTypeStr=int32
  Data Type Conversion1 : DataTypeConversion  Commented=on  OutDataTypeStr=int32
  Gain : Gain  Commented=on  Gain=0.001  OutDataTypeStr=double
  Shift Arithmetic1 : ArithShift  Commented=on  BitShiftNumber=16  BitShiftDirection=Left
  wires:
  Add/1 -> Gain/1
  int_L/1 -> Data Type Conversion/1
  Data Type Conversion/1 -> Add/1
  int_H/1 -> Data Type Conversion1/1
  Data Type Conversion1/1 -> Shift Arithmetic1/1
  Shift Arithmetic1/1 -> Add/2
  Constant/1 -> Data Store Write2/1
  Constant1/1 -> Add1/2
  Add1/1 -> Data Store Write1/1
  Data Store Read/1 -> Add1/1

== system Demo/MotionControl/Reset/Set_P0/eCANA Receive ==
  Bus Selector : BusSelector  Priority=3  OutputSignals=RxWord
  Data Store Read1 : DataStoreRead  DataStoreName=CanMsgA  IndexOptions=Index vector (dialog)  Indices=1  OutputSizes=1
  System Outputs : Subsystem  Priority=2  mask(System Outputs){MailBox=0}
      settings: CopyFcn=cccopyfcn(gcb)  OpenFcn=ccopenfcn('System Outputs Function')
      mask Help: eval('feval(''rtwprivate'',''rtwhelpview'',''rtw_sys_outputs_block'')');
      mask TypeOptions MailBox: 0 | 1 | 2 | 3 | 4 | 5
  DataRx : Outport
  wires:
  Bus Selector/1 -> DataRx/1  "<RxWord>"
  Data Store Read1/1 -> Bus Selector/1

== system Demo/MotionControl/Reset/UM=4/Delay500ms ==

== system Demo/MotionControl/Reset/UM=4/eCANA Transmit ==
  DataTx : Inport
  Bus Assignment : BusAssignment  Priority=1  AssignedSignals=TxWord
  Data Store Read : DataStoreRead  DataStoreName=CanMsgA  IndexOptions=Index vector (dialog)  Indices=1  OutputSizes=1
  Data Store Write : DataStoreWrite  DataStoreName=CanMsgA  IndexOptions=Index vector (dialog)  Indices=1  OutputSizes=1
  System Outputs : Subsystem  Priority=2  mask(System Outputs){MailBox=0}
      settings: CopyFcn=cccopyfcn(gcb)  OpenFcn=ccopenfcn('System Outputs Function')
      mask Help: eval('feval(''rtwprivate'',''rtwhelpview'',''rtw_sys_outputs_block'')');
      mask TypeOptions MailBox: 0 | 1 | 2 | 3 | 4 | 5
  wires:
  DataTx/1 -> Bus Assignment/2
  Data Store Read/1 -> Bus Assignment/1
  Bus Assignment/1 -> Data Store Write/1

== system Demo/MotionControl/Run/Real Motor Control/Enabled Subsystem ==
  Target_AIorTF : Inport
  Enable : EnablePort
  Motor : Outport
  wires:
  Target_AIorTF/1 -> Motor/1

== system Demo/MotionControl/Run/Real Motor Control/Enabled Subsystem1 ==
  Target_AIorTF : Inport
  Enable : EnablePort
  Motor : Outport
  wires:
  Target_AIorTF/1 -> Motor/1

== system Demo/MotionControl/Start/BG/eCANA Transmit ==
  DataTx : Inport
  Bus Assignment : BusAssignment  Priority=1  AssignedSignals=TxWord
  Data Store Read : DataStoreRead  DataStoreName=CanMsgA  IndexOptions=Index vector (dialog)  Indices=1  OutputSizes=1
  Data Store Write : DataStoreWrite  DataStoreName=CanMsgA  IndexOptions=Index vector (dialog)  Indices=1  OutputSizes=1
  System Outputs : Subsystem  Priority=2  mask(System Outputs){MailBox=0}
      settings: CopyFcn=cccopyfcn(gcb)  OpenFcn=ccopenfcn('System Outputs Function')
      mask Help: eval('feval(''rtwprivate'',''rtwhelpview'',''rtw_sys_outputs_block'')');
      mask TypeOptions MailBox: 0 | 1 | 2 | 3 | 4 | 5
  wires:
  Bus Assignment/1 -> Data Store Write/1
  Data Store Read/1 -> Bus Assignment/1
  DataTx/1 -> Bus Assignment/2

== system Demo/MotionControl/Start/MO=1/Delay500ms ==

== system Demo/MotionControl/Start/MO=1/eCANA Transmit ==
  DataTx : Inport
  Bus Assignment : BusAssignment  Priority=1  AssignedSignals=TxWord
  Data Store Read : DataStoreRead  DataStoreName=CanMsgA  IndexOptions=Index vector (dialog)  Indices=1  OutputSizes=1
  Data Store Write : DataStoreWrite  DataStoreName=CanMsgA  IndexOptions=Index vector (dialog)  Indices=1  OutputSizes=1
  System Outputs : Subsystem  Priority=2  mask(System Outputs){MailBox=0}
      settings: CopyFcn=cccopyfcn(gcb)  OpenFcn=ccopenfcn('System Outputs Function')
      mask Help: eval('feval(''rtwprivate'',''rtwhelpview'',''rtw_sys_outputs_block'')');
      mask TypeOptions MailBox: 0 | 1 | 2 | 3 | 4 | 5
  wires:
  DataTx/1 -> Bus Assignment/2
  Data Store Read/1 -> Bus Assignment/1
  Bus Assignment/1 -> Data Store Write/1

== system Demo/MotionControl/Start/UM=1or4/eCANA Transmit ==
  DataTx : Inport
  Bus Assignment : BusAssignment  Priority=1  AssignedSignals=TxWord
  Data Store Read : DataStoreRead  DataStoreName=CanMsgA  IndexOptions=Index vector (dialog)  Indices=1  OutputSizes=1
  Data Store Write : DataStoreWrite  DataStoreName=CanMsgA  IndexOptions=Index vector (dialog)  Indices=1  OutputSizes=1
  System Outputs : Subsystem  Priority=2  mask(System Outputs){MailBox=0}
      settings: CopyFcn=cccopyfcn(gcb)  OpenFcn=ccopenfcn('System Outputs Function')
      mask Help: eval('feval(''rtwprivate'',''rtwhelpview'',''rtw_sys_outputs_block'')');
      mask TypeOptions MailBox: 0 | 1 | 2 | 3 | 4 | 5
  wires:
  Bus Assignment/1 -> Data Store Write/1
  Data Store Read/1 -> Bus Assignment/1
  DataTx/1 -> Bus Assignment/2

== system Demo/Pendulum/Subsystem/CanReceive ==
  Msg : Inport
  Abs : Abs
  Compare To Constant1 : simulink/Logic and Bit Operations/Compare To Constant  relop=<=  const=10  OutDataTypeStr=boolean
  Data Type Conversion3 : DataTypeConversion  OutDataTypeStr=int16
  Demux : Demux
  Gain3 : Gain  Gain=0.01  OutDataTypeStr=double
  Subsystem1 : Subsystem
  wires:
  Msg/1 -> Demux/1
  Demux/1 -> Data Type Conversion3/1
  Abs/1 -> Compare To Constant1/1
  Compare To Constant1/1 -> Subsystem1/Enable
  Data Type Conversion3/1 -> Gain3/1
  Demux/3 -> Subsystem1/2(PosL)
  Demux/4 -> Subsystem1/3(PosH)
  Gain3/1 -> Abs/1, Subsystem1/1(Current)

== system Demo/Pendulum/Subsystem/eCANA Receive ==
  Bus Selector : BusSelector  Priority=3  OutputSignals=RxWord
  Data Store Read1 : DataStoreRead  DataStoreName=CanMsgA  IndexOptions=Index vector (dialog)  Indices=1  OutputSizes=1
  System Outputs : Subsystem  Priority=2  mask(System Outputs){MailBox=0}
      settings: CopyFcn=cccopyfcn(gcb)  OpenFcn=ccopenfcn('System Outputs Function')
      mask Help: eval('feval(''rtwprivate'',''rtwhelpview'',''rtw_sys_outputs_block'')');
      mask TypeOptions MailBox: 0 | 1 | 2 | 3 | 4 | 5
  DataRx : Outport
  wires:
  Bus Selector/1 -> DataRx/1  "<RxWord>"
  Data Store Read1/1 -> Bus Selector/1

== system Demo/Pendulum/Subsystem/eCANA Transmit ==
  DataTx : Inport
  Bus Assignment : BusAssignment  Priority=1  AssignedSignals=TxWord
  Data Store Read : DataStoreRead  DataStoreName=CanMsgA  IndexOptions=Index vector (dialog)  Indices=1  OutputSizes=1
  Data Store Write : DataStoreWrite  DataStoreName=CanMsgA  IndexOptions=Index vector (dialog)  Indices=1  OutputSizes=1
  System Outputs : Subsystem  Priority=2  mask(System Outputs){MailBox=0}
      settings: CopyFcn=cccopyfcn(gcb)  OpenFcn=ccopenfcn('System Outputs Function')
      mask Help: eval('feval(''rtwprivate'',''rtwhelpview'',''rtw_sys_outputs_block'')');
      mask TypeOptions MailBox: 0 | 1 | 2 | 3 | 4 | 5
  wires:
  DataTx/1 -> Bus Assignment/2
  Data Store Read/1 -> Bus Assignment/1
  Bus Assignment/1 -> Data Store Write/1

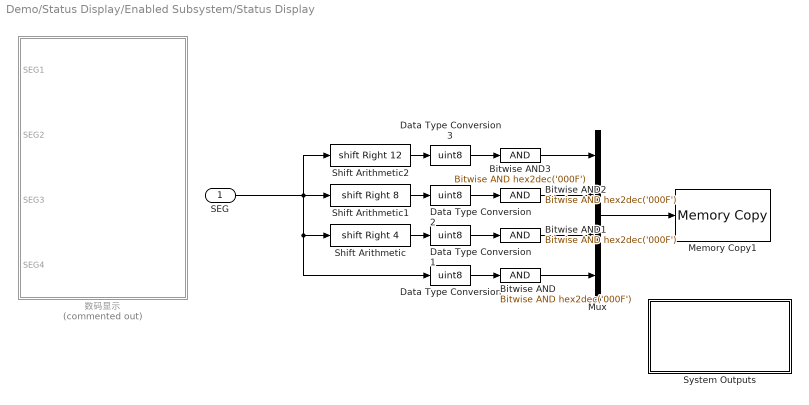
== system Demo/Status Display/Enabled Subsystem/Status Display ==
  SEG : Inport
  Bitwise AND{,1..3} (4 alike) : simulink/Logic and Bit Operations/Bitwise Operator  logicop=AND  UseBitMask=on  BitMask=hex2dec('000F')  BitMaskRealWorld=Stored Integer
  Data Type Conversion{,1..3} (4 alike) : DataTypeConversion  OutDataTypeStr=uint8
  Memory Copy1 : idelinklib_common/Memory Copy  copyFrom=Input port  copyFromAddressSource=Specify via dialog  copyFromAddress=hex2dec('00001000')  copyFromSrcCode=myVariableSrc  dataTypeFrom=uint8  dataDimensionFrom=4  useOffsetFrom=off  offsetFromSrc=Specify via dialog  offsetFrom=0  strideFrom=1  copyTo=Specified source code symbol  copyToAddressSource=Specify via dialog  copyToAddress=hex2dec('00002000')  copyToSrcCode=SEG  dataTypeTo=uint16  useOffsetTo=off  offsetToSrc=Specify via dialog  offsetTo=0  strideTo=1  sampleTime=-1  useInitValue=off  initValueSrc=Specify constant value  initValue=1  initValueSrcCode=myInitValueVariable  useAsMask=off  maskOperator=bitwise AND  useTermValue=off  termValue=1  isRealtimeEnabled=off  emitCCBeforeWrite=off  CCBeforeWrite=/* Custom Code Before Write*/  emitCCAfterWrite=off  CCAfterWrite=/* Custom Code After Write*/  useDMACopy=off  enableBlockingMode=off
      settings: SourceProductBaseCode=ME
  Mux : Mux
  Shift Arithmetic : ArithShift  BitShiftNumber=4  BitShiftDirection=Right
  Shift Arithmetic1 : ArithShift  BitShiftNumber=8  BitShiftDirection=Right
  Shift Arithmetic2 : ArithShift  BitShiftNumber=12  BitShiftDirection=Right
  System Outputs : Subsystem  mask(System Outputs){ShowInLibBrowser=0}
      mask prompts: ShowInLibBrowser "Simulink:masks:CustCodeMaskParam1_MP"
      settings: CopyFcn=cccopyfcn(gcb)  OpenFcn=ccopenfcn('System Outputs Function')
      mask Help: eval('feval(''rtwprivate'',''rtwhelpview'',''rtw_sys_outputs_block'')');
      mask Display: disp('System\nOutputs');
  数码显示 : Subsystem  Commented=on  TreatAsAtomicUnit=on
      mask DialogControl DescGroupVar Prompt: 数码显示
      mask DialogControl DescTextVar Prompt: 从左到右分别为SEG1->SEG4
      mask DialogControl Container3 Prompt: 数值域：
      mask DialogControl Control17 Prompt: [0x00：0x09]表示数值0~9
      mask DialogControl Control18 Prompt: [0x0A：0x0F]表示字符A~F
      mask DialogControl Control19 Prompt: [0x10：0x11]表示全亮~全灭
  wires:
  Mux/1 -> Memory Copy1/1
  Bitwise AND/1 -> Mux/4
  Shift Arithmetic/1 -> Data Type Conversion1/1
  Bitwise AND1/1 -> Mux/3
  Shift Arithmetic1/1 -> Data Type Conversion2/1
  Bitwise AND2/1 -> Mux/2
  Shift Arithmetic2/1 -> Data Type Conversion3/1
  Bitwise AND3/1 -> Mux/1
  SEG/1 -> Shift Arithmetic/1, Data Type Conversion/1, Shift Arithmetic2/1, Shift Arithmetic1/1
  Data Type Conversion/1 -> Bitwise AND/1
  Data Type Conversion1/1 -> Bitwise AND1/1
  Data Type Conversion2/1 -> Bitwise AND2/1
  Data Type Conversion3/1 -> Bitwise AND3/1

== system Demo/Status Display/Enabled Subsystem/Status Display1 ==
  String : Inport
  Bitwise AND{,1..3} (4 alike) : simulink/Logic and Bit Operations/Bitwise Operator  logicop=AND  UseBitMask=on  BitMask=hex2dec('000F')  BitMaskRealWorld=Stored Integer
  Data Type Conversion{,1..3} (4 alike) : DataTypeConversion  OutDataTypeStr=uint8
  Memory Copy1 : idelinklib_common/Memory Copy  copyFrom=Input port  copyFromAddressSource=Specify via dialog  copyFromAddress=hex2dec('00001000')  copyFromSrcCode=myVariableSrc  dataTypeFrom=uint8  dataDimensionFrom=4  useOffsetFrom=off  offsetFromSrc=Specify via dialog  offsetFrom=0  strideFrom=1  copyTo=Specified source code symbol  copyToAddressSource=Specify via dialog  copyToAddress=hex2dec('00002000')  copyToSrcCode=DisplayString1  dataTypeTo=uint8  useOffsetTo=off  offsetToSrc=Specify via dialog  offsetTo=0  strideTo=1  sampleTime=-1  useInitValue=off  initValueSrc=Specify constant value  initValue=1  initValueSrcCode=myInitValueVariable  useAsMask=off  maskOperator=bitwise AND  useTermValue=off  termValue=1  isRealtimeEnabled=off  emitCCBeforeWrite=off  CCBeforeWrite=/* Custom Code Before Write*/  emitCCAfterWrite=off  CCAfterWrite=/* Custom Code After Write*/  useDMACopy=off  enableBlockingMode=off
      settings: SourceProductBaseCode=ME
  Mux : Mux
  Shift Arithmetic : ArithShift  BitShiftNumber=4  BitShiftDirection=Right
  Shift Arithmetic1 : ArithShift  BitShiftNumber=8  BitShiftDirection=Right
  Shift Arithmetic2 : ArithShift  BitShiftNumber=12  BitShiftDirection=Right
  wires:
  Data Type Conversion3/1 -> Bitwise AND3/1
  Data Type Conversion2/1 -> Bitwise AND2/1
  Data Type Conversion1/1 -> Bitwise AND1/1
  Data Type Conversion/1 -> Bitwise AND/1
  String/1 -> Shift Arithmetic1/1, Shift Arithmetic2/1, Data Type Conversion/1, Shift Arithmetic/1
  Bitwise AND3/1 -> Mux/1
  Shift Arithmetic2/1 -> Data Type Conversion3/1
  Bitwise AND2/1 -> Mux/2
  Shift Arithmetic1/1 -> Data Type Conversion2/1
  Bitwise AND1/1 -> Mux/3
  Shift Arithmetic/1 -> Data Type Conversion1/1
  Bitwise AND/1 -> Mux/4
  Mux/1 -> Memory Copy1/1

== system Demo/Status Display/Enabled Subsystem/Status Display2 ==
  String : Inport
  Bitwise AND{,1..3} (4 alike) : simulink/Logic and Bit Operations/Bitwise Operator  logicop=AND  UseBitMask=on  BitMask=hex2dec('000F')  BitMaskRealWorld=Stored Integer
  Data Type Conversion{,1..3} (4 alike) : DataTypeConversion  OutDataTypeStr=uint8
  Memory Copy1 : idelinklib_common/Memory Copy  copyFrom=Input port  copyFromAddressSource=Specify via dialog  copyFromAddress=hex2dec('00001000')  copyFromSrcCode=myVariableSrc  dataTypeFrom=uint8  dataDimensionFrom=4  useOffsetFrom=off  offsetFromSrc=Specify via dialog  offsetFrom=0  strideFrom=1  copyTo=Specified source code symbol  copyToAddressSource=Specify via dialog  copyToAddress=hex2dec('00002000')  copyToSrcCode=DisplayString2  dataTypeTo=uint8  useOffsetTo=off  offsetToSrc=Specify via dialog  offsetTo=0  strideTo=1  sampleTime=-1  useInitValue=off  initValueSrc=Specify constant value  initValue=1  initValueSrcCode=myInitValueVariable  useAsMask=off  maskOperator=bitwise AND  useTermValue=off  termValue=1  isRealtimeEnabled=off  emitCCBeforeWrite=off  CCBeforeWrite=/* Custom Code Before Write*/  emitCCAfterWrite=off  CCAfterWrite=/* Custom Code After Write*/  useDMACopy=off  enableBlockingMode=off
      settings: SourceProductBaseCode=ME
  Mux : Mux
  Shift Arithmetic : ArithShift  BitShiftNumber=4  BitShiftDirection=Right
  Shift Arithmetic1 : ArithShift  BitShiftNumber=8  BitShiftDirection=Right
  Shift Arithmetic2 : ArithShift  BitShiftNumber=12  BitShiftDirection=Right
  wires:
  Mux/1 -> Memory Copy1/1
  Bitwise AND/1 -> Mux/4
  Shift Arithmetic/1 -> Data Type Conversion1/1
  Bitwise AND1/1 -> Mux/3
  Shift Arithmetic1/1 -> Data Type Conversion2/1
  Bitwise AND2/1 -> Mux/2
  Shift Arithmetic2/1 -> Data Type Conversion3/1
  Bitwise AND3/1 -> Mux/1
  String/1 -> Shift Arithmetic/1, Data Type Conversion/1, Shift Arithmetic2/1, Shift Arithmetic1/1
  Data Type Conversion/1 -> Bitwise AND/1
  Data Type Conversion1/1 -> Bitwise AND1/1
  Data Type Conversion2/1 -> Bitwise AND2/1
  Data Type Conversion3/1 -> Bitwise AND3/1

== system Demo/Status Display/Enabled Subsystem/System Outputs1 ==

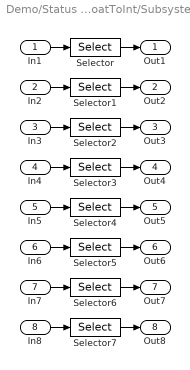
== system Demo/Status Upload/PositionFloatToInt/Subsystem ==
  In1 : Inport
  In2 : Inport  Port=2
  In3 : Inport  Port=3
  In4 : Inport  Port=4
  In5 : Inport  Port=5
  In6 : Inport  Port=6
  In7 : Inport  Port=7
  In8 : Inport  Port=8
  Selector : Selector  InputPortWidth=8  IndexOptions=Index vector (dialog)  Indices=1  OutputSizes=1
  Selector1 : Selector  InputPortWidth=8  IndexOptions=Index vector (dialog)  Indices=2  OutputSizes=1
  Selector2 : Selector  InputPortWidth=8  IndexOptions=Index vector (dialog)  Indices=3  OutputSizes=1
  Selector3 : Selector  InputPortWidth=8  IndexOptions=Index vector (dialog)  Indices=4  OutputSizes=1
  Selector4 : Selector  InputPortWidth=8  IndexOptions=Index vector (dialog)  Indices=5  OutputSizes=1
  Selector5 : Selector  InputPortWidth=8  IndexOptions=Index vector (dialog)  Indices=6  OutputSizes=1
  Selector6 : Selector  InputPortWidth=8  IndexOptions=Index vector (dialog)  Indices=6  OutputSizes=1
  Selector7 : Selector  InputPortWidth=8  IndexOptions=Index vector (dialog)  Indices=6  OutputSizes=1
  Out1 : Outport
  Out2 : Outport  Port=2
  Out3 : Outport  Port=3
  Out4 : Outport  Port=4
  Out5 : Outport  Port=5
  Out6 : Outport  Port=6
  Out7 : Outport  Port=7
  Out8 : Outport  Port=8
  wires:
  In4/1 -> Selector3/1
  Selector4/1 -> Out5/1
  Selector7/1 -> Out8/1
  Selector/1 -> Out1/1
  Selector6/1 -> Out7/1
  In1/1 -> Selector/1
  In8/1 -> Selector7/1
  Selector2/1 -> Out3/1
  Selector1/1 -> Out2/1
  In5/1 -> Selector4/1
  In3/1 -> Selector2/1
  In2/1 -> Selector1/1
  In7/1 -> Selector6/1
  Selector5/1 -> Out6/1
  Selector3/1 -> Out4/1
  In6/1 -> Selector5/1
